simulink model "mass_spring"  (R2018b)
settings: Solver=VariableStepAuto  StartTime=0.0  StopTime=10.0  RelTol=1e-3
undefined symbols (not defined in the file): b, k, m
settings Model: Creator=roberto  LastModifiedBy=roberto

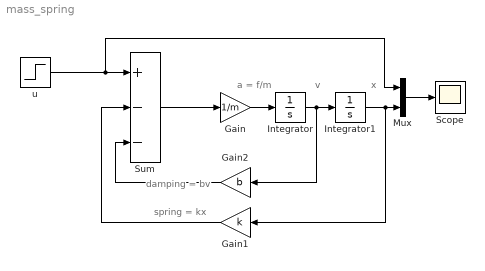
== system mass_spring ==
  note: x
  note: v
  note: a = f/m
  note: spring = kx
  note: damping = bv
  Gain : Gain  Gain=1/m
  Gain1 : Gain  Gain=k
  Gain2 : Gain  Gain=b
  Integrator : Integrator
  Integrator1 : Integrator
  Mux : Mux  Inputs=2
  Scope : Scope
  Sum : Sum  Inputs=+--
  u : Step  SampleTime=0
  wires:
  u/1 -> Mux/1, Sum/1
  Sum/1 -> Gain/1
  Gain/1 -> Integrator/1
  Integrator/1 -> Gain2/1, Integrator1/1
  Integrator1/1 -> Gain1/1, Mux/2
  Mux/1 -> Scope/1
  Gain2/1 -> Sum/3
  Gain1/1 -> Sum/2
